simulink model "UV_sim"  (R2020a)
settings: Solver=FixedStepAuto  StartTime=0.0  StopTime=10.0  FixedStep=0.01  RelTol=1e-3
InitFcn:
  | UV_Parameters;
values from neighbouring files (symbols this model uses):
  p0 = [0,0,0]    [UV_Parameters.m]
  R0 = [cos(psi0)*cos(theta0) -sin(psi0)*cos(theta0)+cos(psi0)*sin(theta0)*sin(phi0) sin(psi0)*sin(phi0)+cos(psi0)*sin(theta0)*cos(phi0);        sin(psi0)*cos(theta0) cos(psi0)*cos(theta0)+sin(psi0)*sin(theta0)*sin(phi0)  -cos(psi0)*sin(phi0)+sin(psi0)*sin(theta0)*cos(phi0);        -sin(theta0)  cos(theta0)*sin(phi0)  cos(theta0)*cos(phi0)]    [UV_Parameters.m]
settings Model: Creator=vcichella  LastModifiedBy=vcichella
settings SFSimCC: CustomCodeUndefinedFunction=UseInterfaceOnly

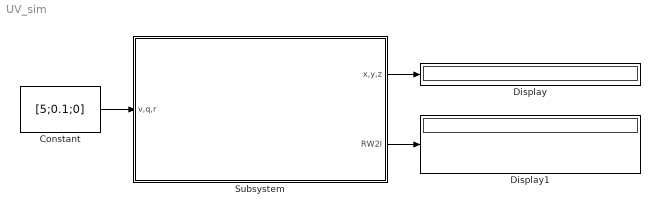
== system UV_sim ==
  Constant : Constant  Value=[5;0.1;0]
  Display : Display
  Display1 : Display
  Subsystem : Subsystem
  wires:
  Constant/1 -> Subsystem/1(v,q,r)
  Subsystem/1(x,y,z) -> Display/1
  Subsystem/2(RW2I) -> Display1/1

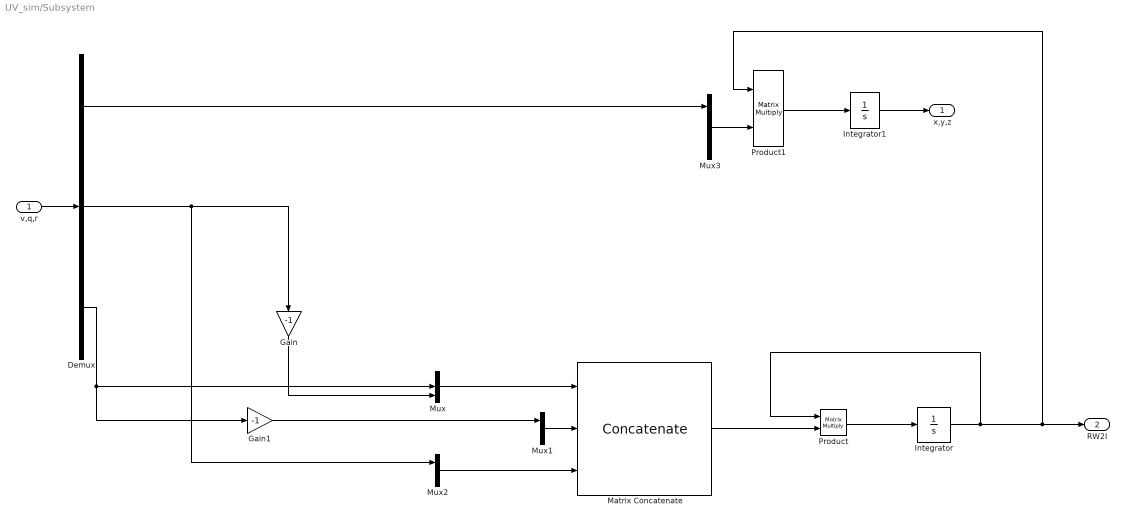
== system UV_sim/Subsystem ==
  v,q,r : Inport
  Demux : Demux  Outputs=3
  Gain : Gain  Gain=-1
  Gain1 : Gain  Gain=-1
  Integrator : Integrator  InitialCondition=R0
  Integrator1 : Integrator  InitialCondition=p0
  Matrix Concatenate : Concatenate  NumInputs=3  Mode=Multidimensional array  ConcatenateDimension=2
  Mux{,1..3} (4 alike) : Mux  Inputs=3
  Product : Product  Multiplication=Matrix(*)
  Product1 : Product  Multiplication=Matrix(*)
  x,y,z : Outport  VectorParamsAs1DForOutWhenUnconnected=off
  RW2I : Outport  Port=2  VectorParamsAs1DForOutWhenUnconnected=off
  wires:
  Matrix Concatenate/1 -> Product/2
  v,q,r/1 -> Demux/1
  Mux/1 -> Matrix Concatenate/1
  Demux/3 -> Gain1/1, Mux/2
  Demux/2 -> Mux2/1, Gain/1
  Gain/1 -> Mux/3
  Mux1/1 -> Matrix Concatenate/2
  Gain1/1 -> Mux1/1
  Mux2/1 -> Matrix Concatenate/3
  Product/1 -> Integrator/1
  Demux/1 -> Mux3/1
  Integrator1/1 -> x,y,z/1
  Product1/1 -> Integrator1/1
  Integrator/1 -> Product1/1, RW2I/1, Product/1
  Mux3/1 -> Product1/2
